simulink library "MyDatacenterModel_GRIDS_HVAC"  (R2025b)
settings: Solver=VariableStepAuto  StartTime=0.0  StopTime=10.0  RelTol=1e-3
libraries: fl_lib x119, datacenter_lib x13, buildingEnergy_lib x11, ee_lib x1
settings Model: Creator=vikrants  LastModifiedBy=skota

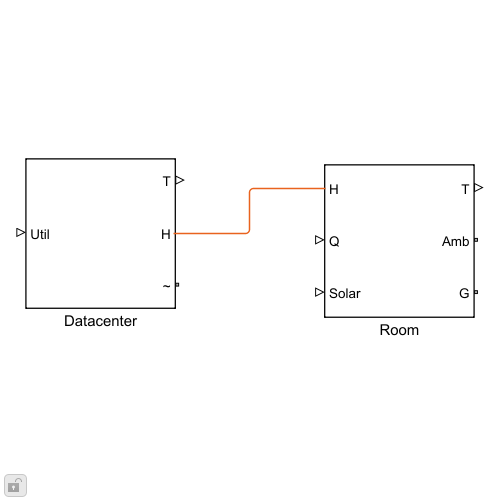
[thumbnail: Simulink's stored preview of the top-level diagram]
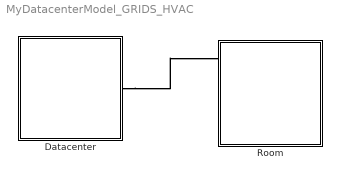
== system MyDatacenterModel_GRIDS_HVAC ==
  Datacenter : Subsystem
  Room : Subsystem
  connections:
  Datacenter/RConn2 -- Room/LConn1

== system MyDatacenterModel_GRIDS_HVAC/Datacenter ==
  Load : ee_lib/Passive/Dynamic Load (Three-Phase)  port_option=ee.enum.threePhasePort.composite  FRated=60 Hz  Vline_rms_min=100 V  tau=0.01 s  Vline_rms_ini=200 V  Vang_ini=0 deg  gmin=0 S
  ServerUnits : Subsystem
  THD : datacenter_lib/Custom Dynamic Load (3-phase) block  Pf=0.98  THD=0  N=12
  Util : PMIOPort  Side=Left
  T : PMIOPort  Port=2  Side=Right
  H : PMIOPort  Port=3  Side=Right
  ~ : PMIOPort  Port=4  Side=Right
  connections:
  ServerUnits/LConn1 -- Util/RConn1
  ServerUnits/RConn2 -- T/RConn1
  ServerUnits/RConn1 -- H/RConn1
  THD/RConn1 -- Load/LConn2
  THD/RConn2 -- Load/LConn3
  THD/LConn1 -- ServerUnits/RConn3
  Load/LConn1 -- ~/RConn1

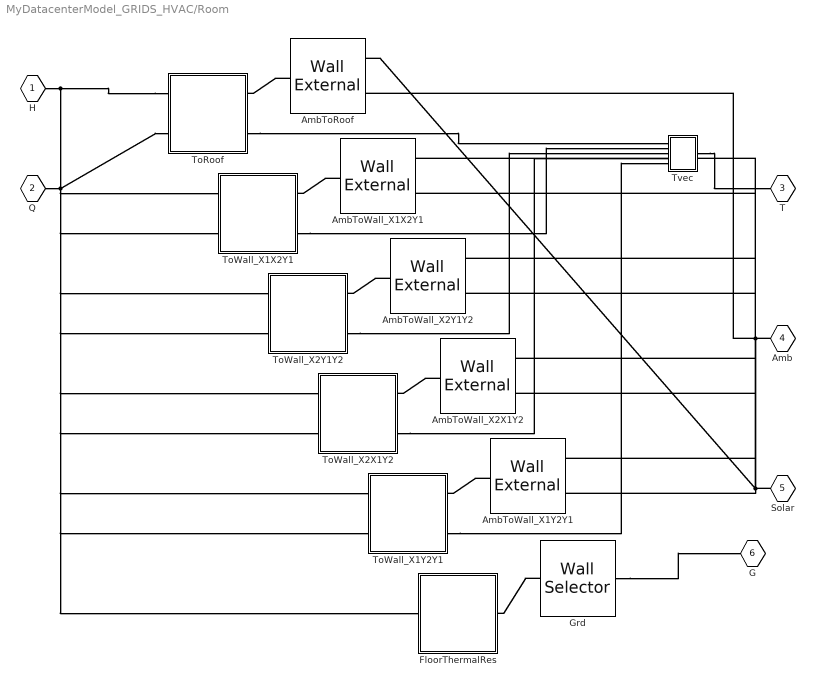
== system MyDatacenterModel_GRIDS_HVAC/Room ==
  AmbToRoof : buildingEnergy_lib/Wall External  extWallModel=wallExternalModelOption.wallSolarWinVent  wallLength=12 m  wallHeight=8 m  wallThickness=0.05 m  wallMaterialDen=4000 kg/m^3  wallMaterialCp=1870 J/(K*kg)  wallAbsorptivity=0.5  wallThermalK=2 W/(K*m)  winLength=1 m  winHeight=0.5 m  winThickness=0.007 m  winMaterialDen=2500 kg/m^3  winMaterialCp=787 J/(K*kg)  winAbsorptivity=0.35  winThermalK=1 W/(K*m)  winTransmissivity=0.45  ventLength=0.1 m  ventHeight=0.1 m  extToWallHTC=5 W/(K*m^2)  intToRoomHTC=5 W/(K*m^2)  iniT=300 K  latitude=5  longitude=5  localTime=5  dayLightS=0  surfAngle=0 deg  surfUnitV="[0.42262    -0.90631]"  startYear=2025  startMonth=1  startDay=1  startHr=1  numHrsData=24  interp_method=simscape.enum.interpolation.linear  extrap_method=simscape.enum.extrapolation.nearest
  AmbToWall_X1X2Y1 : buildingEnergy_lib/Wall External  extWallModel=wallExternalModelOption.wallSolarWinVent  wallLength=12 m  wallHeight=3 m  wallThickness=0.05 m  wallMaterialDen=4000 kg/m^3  wallMaterialCp=1870 J/(K*kg)  wallAbsorptivity=0.5  wallThermalK=2 W/(K*m)  winLength=1 m  winHeight=0.5 m  winThickness=0.007 m  winMaterialDen=2500 kg/m^3  winMaterialCp=787 J/(K*kg)  winAbsorptivity=0.35  winThermalK=1 W/(K*m)  winTransmissivity=0.45  ventLength=0.1 m  ventHeight=0.1 m  extToWallHTC=5 W/(K*m^2)  intToRoomHTC=5 W/(K*m^2)  iniT=300 K  latitude=5  longitude=5  localTime=5  dayLightS=0  surfAngle=90 deg  surfUnitV="[0.42262    -0.90631]"  startYear=2025  startMonth=1  startDay=1  startHr=1  numHrsData=24  interp_method=simscape.enum.interpolation.linear  extrap_method=simscape.enum.extrapolation.nearest
  AmbToWall_X1Y2Y1 : buildingEnergy_lib/Wall External  extWallModel=wallExternalModelOption.wallSolarWinVent  wallLength=8 m  wallHeight=3 m  wallThickness=0.05 m  wallMaterialDen=4000 kg/m^3  wallMaterialCp=1870 J/(K*kg)  wallAbsorptivity=0.5  wallThermalK=2 W/(K*m)  winLength=1 m  winHeight=0.5 m  winThickness=0.007 m  winMaterialDen=2500 kg/m^3  winMaterialCp=787 J/(K*kg)  winAbsorptivity=0.35  winThermalK=1 W/(K*m)  winTransmissivity=0.45  ventLength=0.1 m  ventHeight=0.1 m  extToWallHTC=5 W/(K*m^2)  intToRoomHTC=5 W/(K*m^2)  iniT=300 K  latitude=5  longitude=5  localTime=5  dayLightS=0  surfAngle=90 deg  surfUnitV="[-0.90631    -0.42262]"  startYear=2025  startMonth=1  startDay=1  startHr=1  numHrsData=24  interp_method=simscape.enum.interpolation.linear  extrap_method=simscape.enum.extrapolation.nearest
  AmbToWall_X2X1Y2 : buildingEnergy_lib/Wall External  extWallModel=wallExternalModelOption.wallSolarWinVent  wallLength=12 m  wallHeight=3 m  wallThickness=0.05 m  wallMaterialDen=4000 kg/m^3  wallMaterialCp=1870 J/(K*kg)  wallAbsorptivity=0.5  wallThermalK=2 W/(K*m)  winLength=1 m  winHeight=0.5 m  winThickness=0.007 m  winMaterialDen=2500 kg/m^3  winMaterialCp=787 J/(K*kg)  winAbsorptivity=0.35  winThermalK=1 W/(K*m)  winTransmissivity=0.45  ventLength=0.1 m  ventHeight=0.1 m  extToWallHTC=5 W/(K*m^2)  intToRoomHTC=5 W/(K*m^2)  iniT=300 K  latitude=5  longitude=5  localTime=5  dayLightS=0  surfAngle=90 deg  surfUnitV="[-0.42262     0.90631]"  startYear=2025  startMonth=1  startDay=1  startHr=1  numHrsData=24  interp_method=simscape.enum.interpolation.linear  extrap_method=simscape.enum.extrapolation.nearest
  AmbToWall_X2Y1Y2 : buildingEnergy_lib/Wall External  extWallModel=wallExternalModelOption.wallSolarWinVent  wallLength=8 m  wallHeight=3 m  wallThickness=0.05 m  wallMaterialDen=4000 kg/m^3  wallMaterialCp=1870 J/(K*kg)  wallAbsorptivity=0.5  wallThermalK=2 W/(K*m)  winLength=1 m  winHeight=0.5 m  winThickness=0.007 m  winMaterialDen=2500 kg/m^3  winMaterialCp=787 J/(K*kg)  winAbsorptivity=0.35  winThermalK=1 W/(K*m)  winTransmissivity=0.45  ventLength=0.1 m  ventHeight=0.1 m  extToWallHTC=5 W/(K*m^2)  intToRoomHTC=5 W/(K*m^2)  iniT=300 K  latitude=5  longitude=5  localTime=5  dayLightS=0  surfAngle=90 deg  surfUnitV="[0.90631     0.42262]"  startYear=2025  startMonth=1  startDay=1  startHr=1  numHrsData=24  interp_method=simscape.enum.interpolation.linear  extrap_method=simscape.enum.extrapolation.nearest
  FloorThermalRes : Subsystem
  Grd : buildingEnergy_lib/Wall Selector  optWall=1  wallLength=12 m  wallHeight=8 m  wallThickness=0.05 m  wallMaterialDen=4000 kg/m^3  wallMaterialCp=1870 J/(K*kg)  wallAbsorptivity=0.5  wallThermalK=2 W/(K*m)  winLength=1 m  winHeight=0.5 m  winThickness=0.007 m  winMaterialDen=2500 kg/m^3  winMaterialCp=787 J/(K*kg)  winAbsorptivity=0.35  winThermalK=1 W/(K*m)  winTransmissivity=0.45  ventLength=0.1 m  ventHeight=0.1 m  extToWallHTC=5 W/(K*m^2)  intToRoomHTC=5 W/(K*m^2)  iniT=300 K
  ToRoof : Subsystem
  ToWall_X1X2Y1 : Subsystem
  ToWall_X1Y2Y1 : Subsystem
  ToWall_X2X1Y2 : Subsystem
  ToWall_X2Y1Y2 : Subsystem
  Tvec : Subsystem
  H : PMIOPort  Side=Left
  Q : PMIOPort  Port=2  Side=Left
  T : PMIOPort  Port=3  Side=Right
  Amb : PMIOPort  Port=4  Side=Right
  Solar : PMIOPort  Port=5  Side=Left
  G : PMIOPort  Port=6  Side=Right
  connections:
  ToRoof/LConn1 -- H/RConn1 -- ToWall_X1X2Y1/LConn1 -- ToWall_X2Y1Y2/LConn1 -- ToWall_X2X1Y2/LConn1 -- ToWall_X1Y2Y1/LConn1 -- FloorThermalRes/LConn1
  ToRoof/LConn2 -- Q/RConn1 -- ToWall_X1X2Y1/LConn2 -- ToWall_X2Y1Y2/LConn2 -- ToWall_X2X1Y2/LConn2 -- ToWall_X1Y2Y1/LConn2
  AmbToRoof/RConn1 -- ToRoof/RConn1
  AmbToRoof/LConn2 -- Amb/RConn1 -- AmbToWall_X1X2Y1/LConn2 -- AmbToWall_X2Y1Y2/LConn2 -- AmbToWall_X2X1Y2/LConn2 -- AmbToWall_X1Y2Y1/LConn2
  AmbToRoof/LConn1 -- Solar/RConn1 -- AmbToWall_X1X2Y1/LConn1 -- AmbToWall_X2Y1Y2/LConn1 -- AmbToWall_X2X1Y2/LConn1 -- AmbToWall_X1Y2Y1/LConn1
  ToRoof/RConn2 -- Tvec/LConn1
  AmbToWall_X1X2Y1/RConn1 -- ToWall_X1X2Y1/RConn1
  ToWall_X1X2Y1/RConn2 -- Tvec/LConn2
  AmbToWall_X2Y1Y2/RConn1 -- ToWall_X2Y1Y2/RConn1
  ToWall_X2Y1Y2/RConn2 -- Tvec/LConn3
  AmbToWall_X2X1Y2/RConn1 -- ToWall_X2X1Y2/RConn1
  ToWall_X2X1Y2/RConn2 -- Tvec/LConn4
  AmbToWall_X1Y2Y1/RConn1 -- ToWall_X1Y2Y1/RConn1
  ToWall_X1Y2Y1/RConn2 -- Tvec/LConn5
  Tvec/RConn1 -- T/RConn1
  Grd/LConn1 -- G/RConn1
  Grd/RConn1 -- FloorThermalRes/RConn1

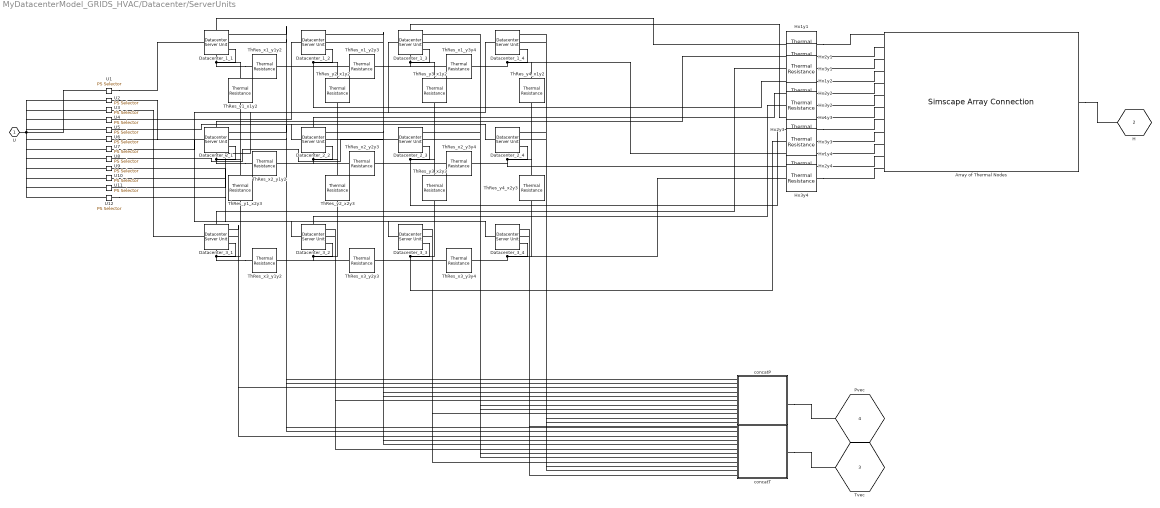
== system MyDatacenterModel_GRIDS_HVAC/Datacenter/ServerUnits ==
  Array of Thermal Nodes : SimscapeArrayConnection  Domain=foundation.thermal.thermal  ConcatenateDimension=1  NumScalarElements=12
  Datacenter_1_{1..4} (4 alike) : datacenter_lib/Datacenter Server Unit  peakPowCPU=40 W  numOfCPU=2  peakPowMemory=9 W  numOfMemory=4  peakPowDisk=12 W  numOfDisk=1  peakPowPCIslot=25 W  numOfPCIslot=2  peakPowMotherboard=25 W  numOfMotherboard=1  peakPowFan=10 W  numOfFan=1  powerSupplyEff=85  numCPUperServer=11  ratioActualToNameplate=0.6  serverMass=50 kg  serverSpHeat=2500 J/(K*kg)  idlePower=25 W  physQ=datacenterPhysics.linear  calibParam=1  T_specify=off  T_priority=High  T=300 K  T_nominal_specify=off  T_nominal_value=1  T_nominal_unit=K  Q_specify=off  Q_priority=None  Q=0 W  Q_nominal_specify=off  Q_nominal_value=1  Q_nominal_unit=W
  Datacenter_2_{1..4} (4 alike) : datacenter_lib/Datacenter Server Unit  peakPowCPU=40 W  numOfCPU=2  peakPowMemory=9 W  numOfMemory=4  peakPowDisk=12 W  numOfDisk=1  peakPowPCIslot=25 W  numOfPCIslot=2  peakPowMotherboard=25 W  numOfMotherboard=1  peakPowFan=10 W  numOfFan=1  powerSupplyEff=85  numCPUperServer=11  ratioActualToNameplate=0.6  serverMass=50 kg  serverSpHeat=2500 J/(K*kg)  idlePower=25 W  physQ=datacenterPhysics.linear  calibParam=1  T_specify=off  T_priority=High  T=300 K  T_nominal_specify=off  T_nominal_value=1  T_nominal_unit=K  Q_specify=off  Q_priority=None  Q=0 W  Q_nominal_specify=off  Q_nominal_value=1  Q_nominal_unit=W
  Datacenter_3_{1..4} (4 alike) : datacenter_lib/Datacenter Server Unit  peakPowCPU=40 W  numOfCPU=2  peakPowMemory=9 W  numOfMemory=4  peakPowDisk=12 W  numOfDisk=1  peakPowPCIslot=25 W  numOfPCIslot=2  peakPowMotherboard=25 W  numOfMotherboard=1  peakPowFan=10 W  numOfFan=1  powerSupplyEff=85  numCPUperServer=11  ratioActualToNameplate=0.6  serverMass=50 kg  serverSpHeat=2500 J/(K*kg)  idlePower=25 W  physQ=datacenterPhysics.linear  calibParam=1  T_specify=off  T_priority=High  T=300 K  T_nominal_specify=off  T_nominal_value=1  T_nominal_unit=K  Q_specify=off  Q_priority=None  Q=0 W  Q_nominal_specify=off  Q_nominal_value=1  Q_nominal_unit=W
  Hx1y{1..4} (4 alike) : fl_lib/Thermal/Thermal Elements/Thermal Resistance  resistance=0.01 K/W  T_specify=off  T_priority=None  T=0 K  T_nominal_specify=off  T_nominal_value=1  T_nominal_unit=K  Q_specify=off  Q_priority=None  Q=0 W  Q_nominal_specify=off  Q_nominal_value=1  Q_nominal_unit=W
  Hx2y{1..4} (4 alike) : fl_lib/Thermal/Thermal Elements/Thermal Resistance  resistance=0.01 K/W  T_specify=off  T_priority=None  T=0 K  T_nominal_specify=off  T_nominal_value=1  T_nominal_unit=K  Q_specify=off  Q_priority=None  Q=0 W  Q_nominal_specify=off  Q_nominal_value=1  Q_nominal_unit=W
  Hx3y{1..4} (4 alike) : fl_lib/Thermal/Thermal Elements/Thermal Resistance  resistance=0.01 K/W  T_specify=off  T_priority=None  T=0 K  T_nominal_specify=off  T_nominal_value=1  T_nominal_unit=K  Q_specify=off  Q_priority=None  Q=0 W  Q_nominal_specify=off  Q_nominal_value=1  Q_nominal_unit=W
  ThRes_x1_y1y2 : fl_lib/Thermal/Thermal Elements/Thermal Resistance  resistance=0.01 K/W  T_specify=off  T_priority=None  T=0 K  T_nominal_specify=off  T_nominal_value=1  T_nominal_unit=K  Q_specify=off  Q_priority=None  Q=0 W  Q_nominal_specify=off  Q_nominal_value=1  Q_nominal_unit=W
  ThRes_x1_y2y3 : fl_lib/Thermal/Thermal Elements/Thermal Resistance  resistance=0.01 K/W  T_specify=off  T_priority=None  T=0 K  T_nominal_specify=off  T_nominal_value=1  T_nominal_unit=K  Q_specify=off  Q_priority=None  Q=0 W  Q_nominal_specify=off  Q_nominal_value=1  Q_nominal_unit=W
  ThRes_x1_y3y4 : fl_lib/Thermal/Thermal Elements/Thermal Resistance  resistance=0.01 K/W  T_specify=off  T_priority=None  T=0 K  T_nominal_specify=off  T_nominal_value=1  T_nominal_unit=K  Q_specify=off  Q_priority=None  Q=0 W  Q_nominal_specify=off  Q_nominal_value=1  Q_nominal_unit=W
  ThRes_x2_y1y2 : fl_lib/Thermal/Thermal Elements/Thermal Resistance  resistance=0.01 K/W  T_specify=off  T_priority=None  T=0 K  T_nominal_specify=off  T_nominal_value=1  T_nominal_unit=K  Q_specify=off  Q_priority=None  Q=0 W  Q_nominal_specify=off  Q_nominal_value=1  Q_nominal_unit=W
  ThRes_x2_y2y3 : fl_lib/Thermal/Thermal Elements/Thermal Resistance  resistance=0.01 K/W  T_specify=off  T_priority=None  T=0 K  T_nominal_specify=off  T_nominal_value=1  T_nominal_unit=K  Q_specify=off  Q_priority=None  Q=0 W  Q_nominal_specify=off  Q_nominal_value=1  Q_nominal_unit=W
  ThRes_x2_y3y4 : fl_lib/Thermal/Thermal Elements/Thermal Resistance  resistance=0.01 K/W  T_specify=off  T_priority=None  T=0 K  T_nominal_specify=off  T_nominal_value=1  T_nominal_unit=K  Q_specify=off  Q_priority=None  Q=0 W  Q_nominal_specify=off  Q_nominal_value=1  Q_nominal_unit=W
  ThRes_x3_y1y2 : fl_lib/Thermal/Thermal Elements/Thermal Resistance  resistance=0.01 K/W  T_specify=off  T_priority=None  T=0 K  T_nominal_specify=off  T_nominal_value=1  T_nominal_unit=K  Q_specify=off  Q_priority=None  Q=0 W  Q_nominal_specify=off  Q_nominal_value=1  Q_nominal_unit=W
  ThRes_x3_y2y3 : fl_lib/Thermal/Thermal Elements/Thermal Resistance  resistance=0.01 K/W  T_specify=off  T_priority=None  T=0 K  T_nominal_specify=off  T_nominal_value=1  T_nominal_unit=K  Q_specify=off  Q_priority=None  Q=0 W  Q_nominal_specify=off  Q_nominal_value=1  Q_nominal_unit=W
  ThRes_x3_y3y4 : fl_lib/Thermal/Thermal Elements/Thermal Resistance  resistance=0.01 K/W  T_specify=off  T_priority=None  T=0 K  T_nominal_specify=off  T_nominal_value=1  T_nominal_unit=K  Q_specify=off  Q_priority=None  Q=0 W  Q_nominal_specify=off  Q_nominal_value=1  Q_nominal_unit=W
  ThRes_y1_x1y2 : fl_lib/Thermal/Thermal Elements/Thermal Resistance  resistance=0.01 K/W  T_specify=off  T_priority=None  T=0 K  T_nominal_specify=off  T_nominal_value=1  T_nominal_unit=K  Q_specify=off  Q_priority=None  Q=0 W  Q_nominal_specify=off  Q_nominal_value=1  Q_nominal_unit=W
  ThRes_y1_x2y3 : fl_lib/Thermal/Thermal Elements/Thermal Resistance  resistance=0.01 K/W  T_specify=off  T_priority=None  T=0 K  T_nominal_specify=off  T_nominal_value=1  T_nominal_unit=K  Q_specify=off  Q_priority=None  Q=0 W  Q_nominal_specify=off  Q_nominal_value=1  Q_nominal_unit=W
  ThRes_y2_x1y2 : fl_lib/Thermal/Thermal Elements/Thermal Resistance  resistance=0.01 K/W  T_specify=off  T_priority=None  T=0 K  T_nominal_specify=off  T_nominal_value=1  T_nominal_unit=K  Q_specify=off  Q_priority=None  Q=0 W  Q_nominal_specify=off  Q_nominal_value=1  Q_nominal_unit=W
  ThRes_y2_x2y3 : fl_lib/Thermal/Thermal Elements/Thermal Resistance  resistance=0.01 K/W  T_specify=off  T_priority=None  T=0 K  T_nominal_specify=off  T_nominal_value=1  T_nominal_unit=K  Q_specify=off  Q_priority=None  Q=0 W  Q_nominal_specify=off  Q_nominal_value=1  Q_nominal_unit=W
  ThRes_y3_x1y2 : fl_lib/Thermal/Thermal Elements/Thermal Resistance  resistance=0.01 K/W  T_specify=off  T_priority=None  T=0 K  T_nominal_specify=off  T_nominal_value=1  T_nominal_unit=K  Q_specify=off  Q_priority=None  Q=0 W  Q_nominal_specify=off  Q_nominal_value=1  Q_nominal_unit=W
  ThRes_y3_x2y3 : fl_lib/Thermal/Thermal Elements/Thermal Resistance  resistance=0.01 K/W  T_specify=off  T_priority=None  T=0 K  T_nominal_specify=off  T_nominal_value=1  T_nominal_unit=K  Q_specify=off  Q_priority=None  Q=0 W  Q_nominal_specify=off  Q_nominal_value=1  Q_nominal_unit=W
  ThRes_y4_x1y2 : fl_lib/Thermal/Thermal Elements/Thermal Resistance  resistance=0.01 K/W  T_specify=off  T_priority=None  T=0 K  T_nominal_specify=off  T_nominal_value=1  T_nominal_unit=K  Q_specify=off  Q_priority=None  Q=0 W  Q_nominal_specify=off  Q_nominal_value=1  Q_nominal_unit=W
  ThRes_y4_x2y3 : fl_lib/Thermal/Thermal Elements/Thermal Resistance  resistance=0.01 K/W  T_specify=off  T_priority=None  T=0 K  T_nominal_specify=off  T_nominal_value=1  T_nominal_unit=K  Q_specify=off  Q_priority=None  Q=0 W  Q_nominal_specify=off  Q_nominal_value=1  Q_nominal_unit=W
  U1 : fl_lib/Physical Signals/Nonlinear Operators/PS Selector  ix=1
  U10 : fl_lib/Physical Signals/Nonlinear Operators/PS Selector  ix=10
  U11 : fl_lib/Physical Signals/Nonlinear Operators/PS Selector  ix=11
  U12 : fl_lib/Physical Signals/Nonlinear Operators/PS Selector  ix=12
  U2 : fl_lib/Physical Signals/Nonlinear Operators/PS Selector  ix=2
  U3 : fl_lib/Physical Signals/Nonlinear Operators/PS Selector  ix=3
  U4 : fl_lib/Physical Signals/Nonlinear Operators/PS Selector  ix=4
  U5 : fl_lib/Physical Signals/Nonlinear Operators/PS Selector  ix=5
  U6 : fl_lib/Physical Signals/Nonlinear Operators/PS Selector  ix=6
  U7 : fl_lib/Physical Signals/Nonlinear Operators/PS Selector  ix=7
  U8 : fl_lib/Physical Signals/Nonlinear Operators/PS Selector  ix=8
  U9 : fl_lib/Physical Signals/Nonlinear Operators/PS Selector  ix=9
  concatP : Subsystem
  concatT : Subsystem
  U : PMIOPort  Side=Left
  H : PMIOPort  Port=2  Side=Right
  Tvec : PMIOPort  Port=3  Side=Right
  Pvec : PMIOPort  Port=4  Side=Right
  connections:
  ThRes_x1_y1y2/LConn1 -- Datacenter_1_1/RConn3 -- ThRes_y1_x1y2/LConn1 -- Hx1y1/LConn1
  ThRes_x1_y1y2/RConn1 -- Datacenter_1_2/RConn3 -- ThRes_x1_y2y3/LConn1 -- ThRes_y2_x1y2/LConn1 -- Hx1y2/LConn1
  ThRes_x1_y2y3/RConn1 -- Datacenter_1_3/RConn3 -- ThRes_x1_y3y4/LConn1 -- ThRes_y3_x1y2/LConn1 -- Hx1y3/LConn1
  ThRes_x1_y3y4/RConn1 -- Datacenter_1_4/RConn3 -- ThRes_y4_x1y2/LConn1 -- Hx1y4/LConn1
  ThRes_x2_y1y2/LConn1 -- Datacenter_2_1/RConn3 -- ThRes_y1_x1y2/RConn1 -- ThRes_y1_x2y3/LConn1 -- Hx2y1/LConn1
  ThRes_x2_y1y2/RConn1 -- Datacenter_2_2/RConn3 -- ThRes_x2_y2y3/LConn1 -- ThRes_y2_x1y2/RConn1 -- ThRes_y2_x2y3/LConn1 -- Hx2y2/LConn1
  ThRes_x2_y2y3/RConn1 -- Datacenter_2_3/RConn3 -- ThRes_x2_y3y4/LConn1 -- ThRes_y3_x1y2/RConn1 -- ThRes_y3_x2y3/LConn1 -- Hx2y3/LConn1
  ThRes_x2_y3y4/RConn1 -- Datacenter_2_4/RConn3 -- ThRes_y4_x1y2/RConn1 -- ThRes_y4_x2y3/LConn1 -- Hx2y4/LConn1
  ThRes_x3_y1y2/LConn1 -- Datacenter_3_1/RConn3 -- ThRes_y1_x2y3/RConn1 -- Hx3y1/LConn1
  ThRes_x3_y1y2/RConn1 -- Datacenter_3_2/RConn3 -- ThRes_x3_y2y3/LConn1 -- ThRes_y2_x2y3/RConn1 -- Hx3y2/LConn1
  ThRes_x3_y2y3/RConn1 -- Datacenter_3_3/RConn3 -- ThRes_x3_y3y4/LConn1 -- ThRes_y3_x2y3/RConn1 -- Hx3y3/LConn1
  ThRes_x3_y3y4/RConn1 -- Datacenter_3_4/RConn3 -- ThRes_y4_x2y3/RConn1 -- Hx3y4/LConn1
  U1/LConn1 -- U2/LConn1 -- U3/LConn1 -- U4/LConn1 -- U5/LConn1 -- U6/LConn1 -- U7/LConn1 -- U8/LConn1 -- U9/LConn1 -- U10/LConn1 -- U11/LConn1 -- U/RConn1 -- U12/LConn1
  U1/RConn1 -- Datacenter_1_1/LConn1
  U2/RConn1 -- Datacenter_2_1/LConn1
  U3/RConn1 -- Datacenter_3_1/LConn1
  U4/RConn1 -- Datacenter_1_2/LConn1
  U5/RConn1 -- Datacenter_2_2/LConn1
  U6/RConn1 -- Datacenter_3_2/LConn1
  U7/RConn1 -- Datacenter_1_3/LConn1
  U8/RConn1 -- Datacenter_2_3/LConn1
  U9/RConn1 -- Datacenter_3_3/LConn1
  U10/RConn1 -- Datacenter_1_4/LConn1
  U11/RConn1 -- Datacenter_2_4/LConn1
  U12/RConn1 -- Datacenter_3_4/LConn1
  Array of Thermal Nodes/RConn1 -- H/RConn1
  Hx1y1/RConn1 -- Array of Thermal Nodes/LConn1
  Hx2y1/RConn1 -- Array of Thermal Nodes/LConn2
  Hx3y1/RConn1 -- Array of Thermal Nodes/LConn3
  Hx1y2/RConn1 -- Array of Thermal Nodes/LConn4
  Hx2y2/RConn1 -- Array of Thermal Nodes/LConn5
  Hx3y2/RConn1 -- Array of Thermal Nodes/LConn6
  Hx1y3/RConn1 -- Array of Thermal Nodes/LConn7
  Hx2y3/RConn1 -- Array of Thermal Nodes/LConn8
  Hx3y3/RConn1 -- Array of Thermal Nodes/LConn9
  Hx1y4/RConn1 -- Array of Thermal Nodes/LConn10
  Hx2y4/RConn1 -- Array of Thermal Nodes/LConn11
  Hx3y4/RConn1 -- Array of Thermal Nodes/LConn12
  concatT/RConn1 -- Tvec/RConn1
  concatT/LConn1 -- Datacenter_1_1/RConn1
  concatT/LConn2 -- Datacenter_2_1/RConn1
  concatT/LConn3 -- Datacenter_3_1/RConn1
  concatT/LConn4 -- Datacenter_1_2/RConn1
  concatT/LConn5 -- Datacenter_2_2/RConn1
  concatT/LConn6 -- Datacenter_3_2/RConn1
  concatT/LConn7 -- Datacenter_1_3/RConn1
  concatT/LConn8 -- Datacenter_2_3/RConn1
  concatT/LConn9 -- Datacenter_3_3/RConn1
  concatT/LConn10 -- Datacenter_1_4/RConn1
  concatT/LConn11 -- Datacenter_2_4/RConn1
  concatT/LConn12 -- Datacenter_3_4/RConn1
  concatP/RConn1 -- Pvec/RConn1
  concatP/LConn1 -- Datacenter_1_1/RConn2
  concatP/LConn2 -- Datacenter_2_1/RConn2
  concatP/LConn3 -- Datacenter_3_1/RConn2
  concatP/LConn4 -- Datacenter_1_2/RConn2
  concatP/LConn5 -- Datacenter_2_2/RConn2
  concatP/LConn6 -- Datacenter_3_2/RConn2
  concatP/LConn7 -- Datacenter_1_3/RConn2
  concatP/LConn8 -- Datacenter_2_3/RConn2
  concatP/LConn9 -- Datacenter_3_3/RConn2
  concatP/LConn10 -- Datacenter_1_4/RConn2
  concatP/LConn11 -- Datacenter_2_4/RConn2
  concatP/LConn12 -- Datacenter_3_4/RConn2

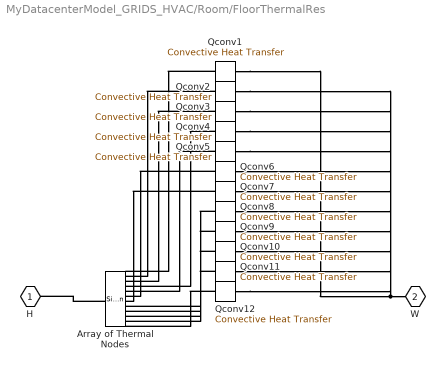
== system MyDatacenterModel_GRIDS_HVAC/Room/FloorThermalRes ==
  Array of Thermal Nodes : SimscapeArrayConnection  Domain=foundation.thermal.thermal  ConcatenateDimension=1  NumScalarElements=12
  Qconv{1..12} (12 alike) : fl_lib/Thermal/Thermal Elements/Convective Heat Transfer  thermal_type=foundation.enum.constant_variable.constant  area=8 m^2  heat_tr_coeff=20 W/(K*m^2)  min_heat_tr_coeff=1e-3 W/(K*m^2)  T_specify=off  T_priority=None  T=0 K  T_nominal_specify=off  T_nominal_value=1  T_nominal_unit=K  Q_specify=off  Q_priority=None  Q=0 W  Q_nominal_specify=off  Q_nominal_value=1  Q_nominal_unit=W
  H : PMIOPort  Side=Left
  W : PMIOPort  Port=2  Side=Right
  connections:
  Array of Thermal Nodes/RConn1 -- H/RConn1
  Qconv1/LConn1 -- Array of Thermal Nodes/LConn1
  Qconv1/RConn1 -- Qconv2/RConn1 -- Qconv3/RConn1 -- Qconv4/RConn1 -- Qconv5/RConn1 -- Qconv6/RConn1 -- Qconv7/RConn1 -- Qconv8/RConn1 -- Qconv9/RConn1 -- Qconv10/RConn1 -- Qconv11/RConn1 -- W/RConn1 -- Qconv12/RConn1
  Qconv2/LConn1 -- Array of Thermal Nodes/LConn2
  Qconv3/LConn1 -- Array of Thermal Nodes/LConn3
  Qconv4/LConn1 -- Array of Thermal Nodes/LConn4
  Qconv5/LConn1 -- Array of Thermal Nodes/LConn5
  Qconv6/LConn1 -- Array of Thermal Nodes/LConn6
  Qconv7/LConn1 -- Array of Thermal Nodes/LConn7
  Qconv8/LConn1 -- Array of Thermal Nodes/LConn8
  Qconv9/LConn1 -- Array of Thermal Nodes/LConn9
  Qconv10/LConn1 -- Array of Thermal Nodes/LConn10
  Qconv11/LConn1 -- Array of Thermal Nodes/LConn11
  Qconv12/LConn1 -- Array of Thermal Nodes/LConn12

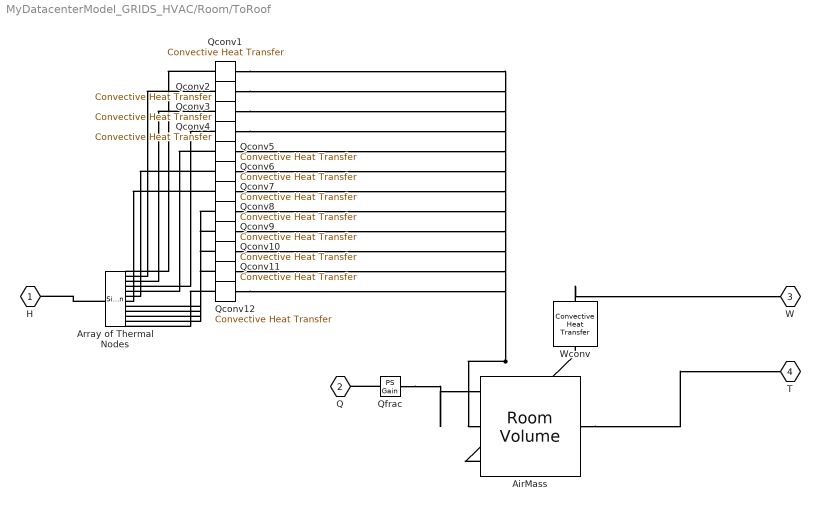
== system MyDatacenterModel_GRIDS_HVAC/Room/ToRoof ==
  AirMass : buildingEnergy_lib/Room Volume  N1=1  N2=1  iniT=300 K  length=12 m  width=8 m  height=0.10667 m
  Array of Thermal Nodes : SimscapeArrayConnection  Domain=foundation.thermal.thermal  ConcatenateDimension=1  NumScalarElements=12
  Qconv{1..12} (12 alike) : fl_lib/Thermal/Thermal Elements/Convective Heat Transfer  thermal_type=foundation.enum.constant_variable.constant  area=8 m^2  heat_tr_coeff=20 W/(K*m^2)  min_heat_tr_coeff=1e-3 W/(K*m^2)  T_specify=off  T_priority=None  T=0 K  T_nominal_specify=off  T_nominal_value=1  T_nominal_unit=K  Q_specify=off  Q_priority=None  Q=0 W  Q_nominal_specify=off  Q_nominal_value=1  Q_nominal_unit=W
  Qfrac : fl_lib/Physical Signals/Functions/PS Gain  gain=0.44444
  Wconv : fl_lib/Thermal/Thermal Elements/Convective Heat Transfer  thermal_type=foundation.enum.constant_variable.constant  area=96 m^2  heat_tr_coeff=20 W/(K*m^2)  min_heat_tr_coeff=1e-3 W/(K*m^2)  T_specify=off  T_priority=None  T=0 K  T_nominal_specify=off  T_nominal_value=1  T_nominal_unit=K  Q_specify=off  Q_priority=None  Q=0 W  Q_nominal_specify=off  Q_nominal_value=1  Q_nominal_unit=W
  H : PMIOPort  Side=Left
  Q : PMIOPort  Port=2  Side=Left
  W : PMIOPort  Port=3  Side=Right
  T : PMIOPort  Port=4  Side=Right
  connections:
  Array of Thermal Nodes/RConn1 -- H/RConn1
  Qfrac/LConn1 -- Q/RConn1
  Qfrac/RConn1 -- AirMass/LConn1
  AirMass/LConn3 -- Wconv/LConn1
  Wconv/RConn1 -- W/RConn1
  AirMass/RConn1 -- T/RConn1
  Qconv1/LConn1 -- Array of Thermal Nodes/LConn1
  Qconv1/RConn1 -- Qconv2/RConn1 -- Qconv3/RConn1 -- Qconv4/RConn1 -- Qconv5/RConn1 -- Qconv6/RConn1 -- Qconv7/RConn1 -- Qconv8/RConn1 -- Qconv9/RConn1 -- Qconv10/RConn1 -- Qconv11/RConn1 -- AirMass/LConn2 -- Qconv12/RConn1
  Qconv2/LConn1 -- Array of Thermal Nodes/LConn2
  Qconv3/LConn1 -- Array of Thermal Nodes/LConn3
  Qconv4/LConn1 -- Array of Thermal Nodes/LConn4
  Qconv5/LConn1 -- Array of Thermal Nodes/LConn5
  Qconv6/LConn1 -- Array of Thermal Nodes/LConn6
  Qconv7/LConn1 -- Array of Thermal Nodes/LConn7
  Qconv8/LConn1 -- Array of Thermal Nodes/LConn8
  Qconv9/LConn1 -- Array of Thermal Nodes/LConn9
  Qconv10/LConn1 -- Array of Thermal Nodes/LConn10
  Qconv11/LConn1 -- Array of Thermal Nodes/LConn11
  Qconv12/LConn1 -- Array of Thermal Nodes/LConn12

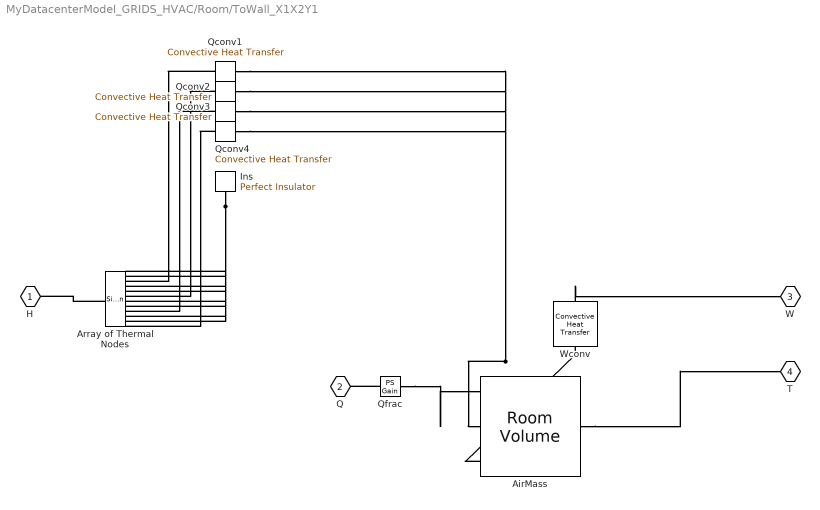
== system MyDatacenterModel_GRIDS_HVAC/Room/ToWall_X1X2Y1 ==
  AirMass : buildingEnergy_lib/Room Volume  N1=1  N2=1  iniT=300 K  length=12 m  width=0.10667 m  height=8 m
  Array of Thermal Nodes : SimscapeArrayConnection  Domain=foundation.thermal.thermal  ConcatenateDimension=1  NumScalarElements=12
  Ins : fl_lib/Thermal/Thermal Elements/Perfect Insulator  T_specify=off  T_priority=None  T=293.15 K  T_nominal_specify=off  T_nominal_value=1  T_nominal_unit=K
  Qconv{1..4} (4 alike) : fl_lib/Thermal/Thermal Elements/Convective Heat Transfer  thermal_type=foundation.enum.constant_variable.constant  area=12 m^2  heat_tr_coeff=20 W/(K*m^2)  min_heat_tr_coeff=1e-3 W/(K*m^2)  T_specify=off  T_priority=None  T=0 K  T_nominal_specify=off  T_nominal_value=1  T_nominal_unit=K  Q_specify=off  Q_priority=None  Q=0 W  Q_nominal_specify=off  Q_nominal_value=1  Q_nominal_unit=W
  Qfrac : fl_lib/Physical Signals/Functions/PS Gain  gain=0.16667
  Wconv : fl_lib/Thermal/Thermal Elements/Convective Heat Transfer  thermal_type=foundation.enum.constant_variable.constant  area=36 m^2  heat_tr_coeff=20 W/(K*m^2)  min_heat_tr_coeff=1e-3 W/(K*m^2)  T_specify=off  T_priority=None  T=0 K  T_nominal_specify=off  T_nominal_value=1  T_nominal_unit=K  Q_specify=off  Q_priority=None  Q=0 W  Q_nominal_specify=off  Q_nominal_value=1  Q_nominal_unit=W
  H : PMIOPort  Side=Left
  Q : PMIOPort  Port=2  Side=Left
  W : PMIOPort  Port=3  Side=Right
  T : PMIOPort  Port=4  Side=Right
  connections:
  Array of Thermal Nodes/RConn1 -- H/RConn1
  Qfrac/LConn1 -- Q/RConn1
  Qfrac/RConn1 -- AirMass/LConn1
  AirMass/LConn3 -- Wconv/LConn1
  Wconv/RConn1 -- W/RConn1
  AirMass/RConn1 -- T/RConn1
  Qconv1/LConn1 -- Array of Thermal Nodes/LConn3
  Qconv1/RConn1 -- Qconv2/RConn1 -- Qconv3/RConn1 -- AirMass/LConn2 -- Qconv4/RConn1
  Qconv2/LConn1 -- Array of Thermal Nodes/LConn6
  Qconv3/LConn1 -- Array of Thermal Nodes/LConn9
  Qconv4/LConn1 -- Array of Thermal Nodes/LConn12
  Array of Thermal Nodes/LConn1 -- Ins/LConn1 -- Array of Thermal Nodes/LConn2 -- Array of Thermal Nodes/LConn4 -- Array of Thermal Nodes/LConn5 -- Array of Thermal Nodes/LConn7 -- Array of Thermal Nodes/LConn8 -- Array of Thermal Nodes/LConn10 -- Array of Thermal Nodes/LConn11

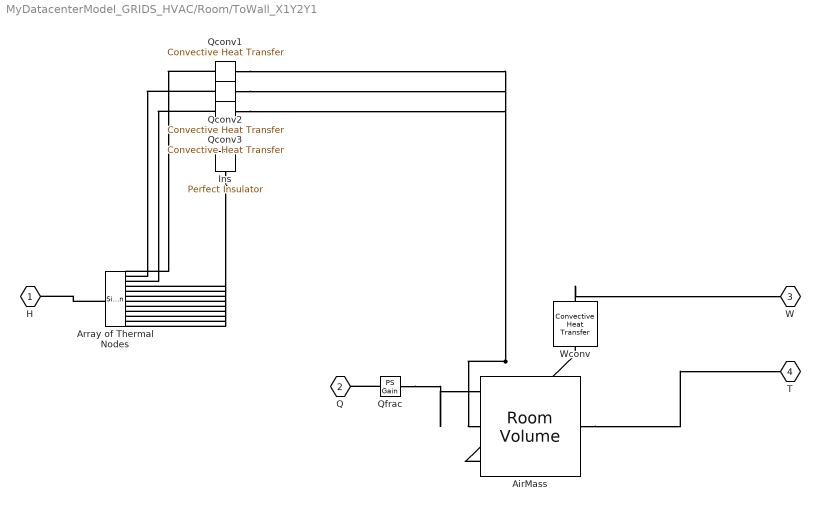
== system MyDatacenterModel_GRIDS_HVAC/Room/ToWall_X1Y2Y1 ==
  AirMass : buildingEnergy_lib/Room Volume  N1=1  N2=1  iniT=300 K  length=8 m  width=0.10667 m  height=3 m
  Array of Thermal Nodes : SimscapeArrayConnection  Domain=foundation.thermal.thermal  ConcatenateDimension=1  NumScalarElements=12
  Ins : fl_lib/Thermal/Thermal Elements/Perfect Insulator  T_specify=off  T_priority=None  T=293.15 K  T_nominal_specify=off  T_nominal_value=1  T_nominal_unit=K
  Qconv1 : fl_lib/Thermal/Thermal Elements/Convective Heat Transfer  thermal_type=foundation.enum.constant_variable.constant  area=6 m^2  heat_tr_coeff=20 W/(K*m^2)  min_heat_tr_coeff=1e-3 W/(K*m^2)  T_specify=off  T_priority=None  T=0 K  T_nominal_specify=off  T_nominal_value=1  T_nominal_unit=K  Q_specify=off  Q_priority=None  Q=0 W  Q_nominal_specify=off  Q_nominal_value=1  Q_nominal_unit=W
  Qconv2 : fl_lib/Thermal/Thermal Elements/Convective Heat Transfer  thermal_type=foundation.enum.constant_variable.constant  area=6 m^2  heat_tr_coeff=20 W/(K*m^2)  min_heat_tr_coeff=1e-3 W/(K*m^2)  T_specify=off  T_priority=None  T=0 K  T_nominal_specify=off  T_nominal_value=1  T_nominal_unit=K  Q_specify=off  Q_priority=None  Q=0 W  Q_nominal_specify=off  Q_nominal_value=1  Q_nominal_unit=W
  Qconv3 : fl_lib/Thermal/Thermal Elements/Convective Heat Transfer  thermal_type=foundation.enum.constant_variable.constant  area=6 m^2  heat_tr_coeff=20 W/(K*m^2)  min_heat_tr_coeff=1e-3 W/(K*m^2)  T_specify=off  T_priority=None  T=0 K  T_nominal_specify=off  T_nominal_value=1  T_nominal_unit=K  Q_specify=off  Q_priority=None  Q=0 W  Q_nominal_specify=off  Q_nominal_value=1  Q_nominal_unit=W
  Qfrac : fl_lib/Physical Signals/Functions/PS Gain  gain=0.11111
  Wconv : fl_lib/Thermal/Thermal Elements/Convective Heat Transfer  thermal_type=foundation.enum.constant_variable.constant  area=24 m^2  heat_tr_coeff=20 W/(K*m^2)  min_heat_tr_coeff=1e-3 W/(K*m^2)  T_specify=off  T_priority=None  T=0 K  T_nominal_specify=off  T_nominal_value=1  T_nominal_unit=K  Q_specify=off  Q_priority=None  Q=0 W  Q_nominal_specify=off  Q_nominal_value=1  Q_nominal_unit=W
  H : PMIOPort  Side=Left
  Q : PMIOPort  Port=2  Side=Left
  W : PMIOPort  Port=3  Side=Right
  T : PMIOPort  Port=4  Side=Right
  connections:
  Array of Thermal Nodes/RConn1 -- H/RConn1
  Qfrac/LConn1 -- Q/RConn1
  Qfrac/RConn1 -- AirMass/LConn1
  AirMass/LConn3 -- Wconv/LConn1
  Wconv/RConn1 -- W/RConn1
  AirMass/RConn1 -- T/RConn1
  Qconv1/LConn1 -- Array of Thermal Nodes/LConn1
  Qconv1/RConn1 -- Qconv2/RConn1 -- AirMass/LConn2 -- Qconv3/RConn1
  Qconv2/LConn1 -- Array of Thermal Nodes/LConn2
  Qconv3/LConn1 -- Array of Thermal Nodes/LConn3
  Array of Thermal Nodes/LConn4 -- Ins/LConn1 -- Array of Thermal Nodes/LConn5 -- Array of Thermal Nodes/LConn6 -- Array of Thermal Nodes/LConn7 -- Array of Thermal Nodes/LConn8 -- Array of Thermal Nodes/LConn9 -- Array of Thermal Nodes/LConn10 -- Array of Thermal Nodes/LConn11 -- Array of Thermal Nodes/LConn12

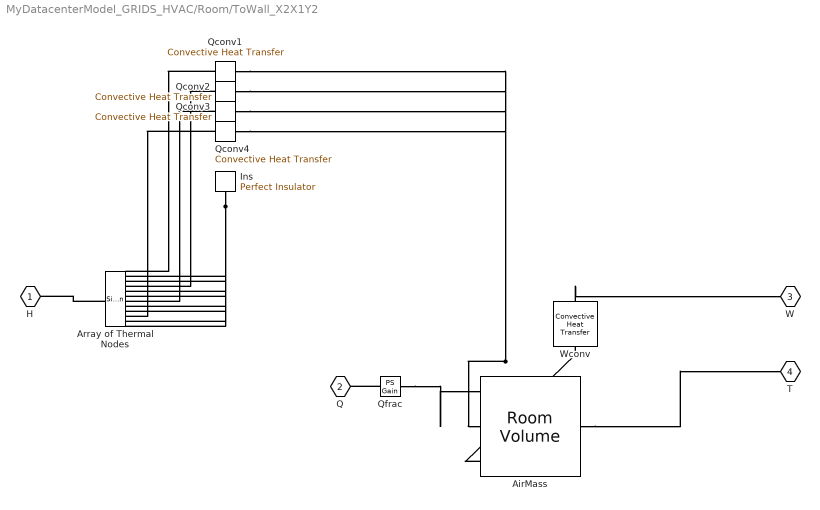
== system MyDatacenterModel_GRIDS_HVAC/Room/ToWall_X2X1Y2 ==
  AirMass : buildingEnergy_lib/Room Volume  N1=1  N2=1  iniT=300 K  length=12 m  width=0.10667 m  height=3 m
  Array of Thermal Nodes : SimscapeArrayConnection  Domain=foundation.thermal.thermal  ConcatenateDimension=1  NumScalarElements=12
  Ins : fl_lib/Thermal/Thermal Elements/Perfect Insulator  T_specify=off  T_priority=None  T=293.15 K  T_nominal_specify=off  T_nominal_value=1  T_nominal_unit=K
  Qconv{1..4} (4 alike) : fl_lib/Thermal/Thermal Elements/Convective Heat Transfer  thermal_type=foundation.enum.constant_variable.constant  area=12 m^2  heat_tr_coeff=20 W/(K*m^2)  min_heat_tr_coeff=1e-3 W/(K*m^2)  T_specify=off  T_priority=None  T=0 K  T_nominal_specify=off  T_nominal_value=1  T_nominal_unit=K  Q_specify=off  Q_priority=None  Q=0 W  Q_nominal_specify=off  Q_nominal_value=1  Q_nominal_unit=W
  Qfrac : fl_lib/Physical Signals/Functions/PS Gain  gain=0.16667
  Wconv : fl_lib/Thermal/Thermal Elements/Convective Heat Transfer  thermal_type=foundation.enum.constant_variable.constant  area=36 m^2  heat_tr_coeff=20 W/(K*m^2)  min_heat_tr_coeff=1e-3 W/(K*m^2)  T_specify=off  T_priority=None  T=0 K  T_nominal_specify=off  T_nominal_value=1  T_nominal_unit=K  Q_specify=off  Q_priority=None  Q=0 W  Q_nominal_specify=off  Q_nominal_value=1  Q_nominal_unit=W
  H : PMIOPort  Side=Left
  Q : PMIOPort  Port=2  Side=Left
  W : PMIOPort  Port=3  Side=Right
  T : PMIOPort  Port=4  Side=Right
  connections:
  Array of Thermal Nodes/RConn1 -- H/RConn1
  Qfrac/LConn1 -- Q/RConn1
  Qfrac/RConn1 -- AirMass/LConn1
  AirMass/LConn3 -- Wconv/LConn1
  Wconv/RConn1 -- W/RConn1
  AirMass/RConn1 -- T/RConn1
  Qconv1/LConn1 -- Array of Thermal Nodes/LConn1
  Qconv1/RConn1 -- Qconv2/RConn1 -- Qconv3/RConn1 -- AirMass/LConn2 -- Qconv4/RConn1
  Qconv2/LConn1 -- Array of Thermal Nodes/LConn4
  Qconv3/LConn1 -- Array of Thermal Nodes/LConn7
  Qconv4/LConn1 -- Array of Thermal Nodes/LConn10
  Array of Thermal Nodes/LConn2 -- Ins/LConn1 -- Array of Thermal Nodes/LConn3 -- Array of Thermal Nodes/LConn5 -- Array of Thermal Nodes/LConn6 -- Array of Thermal Nodes/LConn8 -- Array of Thermal Nodes/LConn9 -- Array of Thermal Nodes/LConn11 -- Array of Thermal Nodes/LConn12

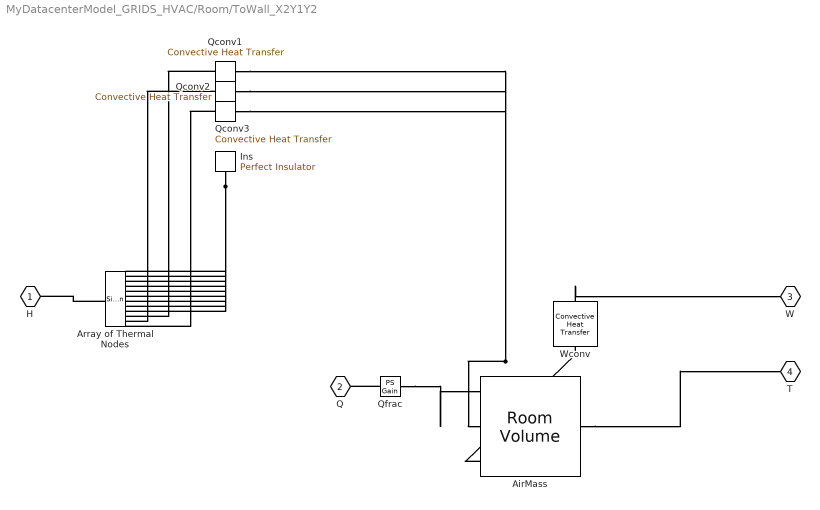
== system MyDatacenterModel_GRIDS_HVAC/Room/ToWall_X2Y1Y2 ==
  AirMass : buildingEnergy_lib/Room Volume  N1=1  N2=1  iniT=300 K  length=8 m  width=0.10667 m  height=3 m
  Array of Thermal Nodes : SimscapeArrayConnection  Domain=foundation.thermal.thermal  ConcatenateDimension=1  NumScalarElements=12
  Ins : fl_lib/Thermal/Thermal Elements/Perfect Insulator  T_specify=off  T_priority=None  T=293.15 K  T_nominal_specify=off  T_nominal_value=1  T_nominal_unit=K
  Qconv1 : fl_lib/Thermal/Thermal Elements/Convective Heat Transfer  thermal_type=foundation.enum.constant_variable.constant  area=6 m^2  heat_tr_coeff=20 W/(K*m^2)  min_heat_tr_coeff=1e-3 W/(K*m^2)  T_specify=off  T_priority=None  T=0 K  T_nominal_specify=off  T_nominal_value=1  T_nominal_unit=K  Q_specify=off  Q_priority=None  Q=0 W  Q_nominal_specify=off  Q_nominal_value=1  Q_nominal_unit=W
  Qconv2 : fl_lib/Thermal/Thermal Elements/Convective Heat Transfer  thermal_type=foundation.enum.constant_variable.constant  area=6 m^2  heat_tr_coeff=20 W/(K*m^2)  min_heat_tr_coeff=1e-3 W/(K*m^2)  T_specify=off  T_priority=None  T=0 K  T_nominal_specify=off  T_nominal_value=1  T_nominal_unit=K  Q_specify=off  Q_priority=None  Q=0 W  Q_nominal_specify=off  Q_nominal_value=1  Q_nominal_unit=W
  Qconv3 : fl_lib/Thermal/Thermal Elements/Convective Heat Transfer  thermal_type=foundation.enum.constant_variable.constant  area=6 m^2  heat_tr_coeff=20 W/(K*m^2)  min_heat_tr_coeff=1e-3 W/(K*m^2)  T_specify=off  T_priority=None  T=0 K  T_nominal_specify=off  T_nominal_value=1  T_nominal_unit=K  Q_specify=off  Q_priority=None  Q=0 W  Q_nominal_specify=off  Q_nominal_value=1  Q_nominal_unit=W
  Qfrac : fl_lib/Physical Signals/Functions/PS Gain  gain=0.11111
  Wconv : fl_lib/Thermal/Thermal Elements/Convective Heat Transfer  thermal_type=foundation.enum.constant_variable.constant  area=24 m^2  heat_tr_coeff=20 W/(K*m^2)  min_heat_tr_coeff=1e-3 W/(K*m^2)  T_specify=off  T_priority=None  T=0 K  T_nominal_specify=off  T_nominal_value=1  T_nominal_unit=K  Q_specify=off  Q_priority=None  Q=0 W  Q_nominal_specify=off  Q_nominal_value=1  Q_nominal_unit=W
  H : PMIOPort  Side=Left
  Q : PMIOPort  Port=2  Side=Left
  W : PMIOPort  Port=3  Side=Right
  T : PMIOPort  Port=4  Side=Right
  connections:
  Array of Thermal Nodes/RConn1 -- H/RConn1
  Qfrac/LConn1 -- Q/RConn1
  Qfrac/RConn1 -- AirMass/LConn1
  AirMass/LConn3 -- Wconv/LConn1
  Wconv/RConn1 -- W/RConn1
  AirMass/RConn1 -- T/RConn1
  Qconv1/LConn1 -- Array of Thermal Nodes/LConn10
  Qconv1/RConn1 -- Qconv2/RConn1 -- AirMass/LConn2 -- Qconv3/RConn1
  Qconv2/LConn1 -- Array of Thermal Nodes/LConn11
  Qconv3/LConn1 -- Array of Thermal Nodes/LConn12
  Array of Thermal Nodes/LConn1 -- Ins/LConn1 -- Array of Thermal Nodes/LConn2 -- Array of Thermal Nodes/LConn3 -- Array of Thermal Nodes/LConn4 -- Array of Thermal Nodes/LConn5 -- Array of Thermal Nodes/LConn6 -- Array of Thermal Nodes/LConn7 -- Array of Thermal Nodes/LConn8 -- Array of Thermal Nodes/LConn9

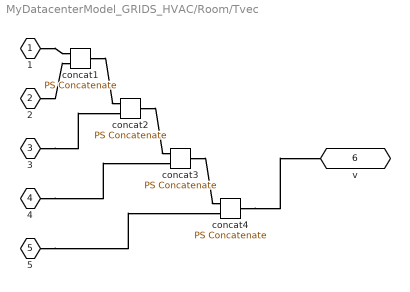
== system MyDatacenterModel_GRIDS_HVAC/Room/Tvec ==
  concat{1..4} (4 alike) : fl_lib/Physical Signals/Functions/PS Concatenate  catColumns=true
  1 : PMIOPort  Side=Left
  2 : PMIOPort  Port=2  Side=Left
  3 : PMIOPort  Port=3  Side=Left
  4 : PMIOPort  Port=4  Side=Left
  5 : PMIOPort  Port=5  Side=Left
  v : PMIOPort  Port=6  Side=Right
  connections:
  1/RConn1 -- concat1/LConn1
  2/RConn1 -- concat1/LConn2
  concat1/RConn1 -- concat2/LConn1
  3/RConn1 -- concat2/LConn2
  concat2/RConn1 -- concat3/LConn1
  4/RConn1 -- concat3/LConn2
  concat3/RConn1 -- concat4/LConn1
  5/RConn1 -- concat4/LConn2
  concat4/RConn1 -- v/RConn1

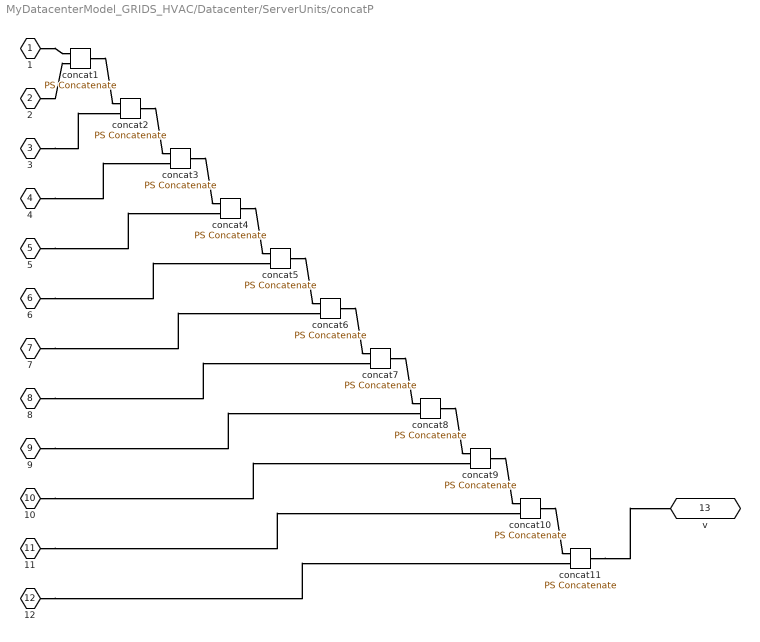
== system MyDatacenterModel_GRIDS_HVAC/Datacenter/ServerUnits/concatP ==
  concat{1..11} (11 alike) : fl_lib/Physical Signals/Functions/PS Concatenate  catColumns=true
  1 : PMIOPort  Side=Left
  2 : PMIOPort  Port=2  Side=Left
  3 : PMIOPort  Port=3  Side=Left
  4 : PMIOPort  Port=4  Side=Left
  5 : PMIOPort  Port=5  Side=Left
  6 : PMIOPort  Port=6  Side=Left
  7 : PMIOPort  Port=7  Side=Left
  8 : PMIOPort  Port=8  Side=Left
  9 : PMIOPort  Port=9  Side=Left
  10 : PMIOPort  Port=10  Side=Left
  11 : PMIOPort  Port=11  Side=Left
  12 : PMIOPort  Port=12  Side=Left
  v : PMIOPort  Port=13  Side=Right
  connections:
  1/RConn1 -- concat1/LConn1
  2/RConn1 -- concat1/LConn2
  concat1/RConn1 -- concat2/LConn1
  3/RConn1 -- concat2/LConn2
  concat2/RConn1 -- concat3/LConn1
  4/RConn1 -- concat3/LConn2
  concat3/RConn1 -- concat4/LConn1
  5/RConn1 -- concat4/LConn2
  concat4/RConn1 -- concat5/LConn1
  6/RConn1 -- concat5/LConn2
  concat5/RConn1 -- concat6/LConn1
  7/RConn1 -- concat6/LConn2
  concat6/RConn1 -- concat7/LConn1
  8/RConn1 -- concat7/LConn2
  concat7/RConn1 -- concat8/LConn1
  9/RConn1 -- concat8/LConn2
  concat8/RConn1 -- concat9/LConn1
  10/RConn1 -- concat9/LConn2
  concat9/RConn1 -- concat10/LConn1
  11/RConn1 -- concat10/LConn2
  concat10/RConn1 -- concat11/LConn1
  12/RConn1 -- concat11/LConn2
  concat11/RConn1 -- v/RConn1

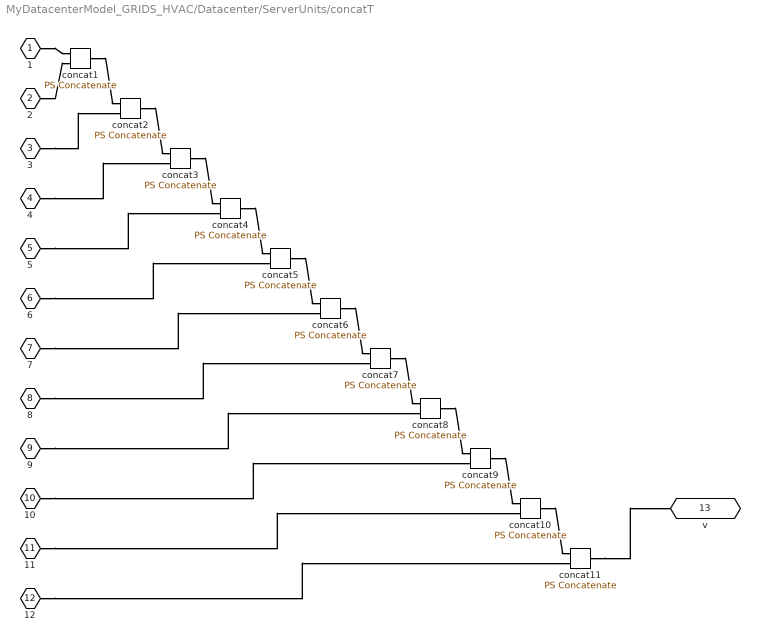
== system MyDatacenterModel_GRIDS_HVAC/Datacenter/ServerUnits/concatT ==
  concat{1..11} (11 alike) : fl_lib/Physical Signals/Functions/PS Concatenate  catColumns=true
  1 : PMIOPort  Side=Left
  2 : PMIOPort  Port=2  Side=Left
  3 : PMIOPort  Port=3  Side=Left
  4 : PMIOPort  Port=4  Side=Left
  5 : PMIOPort  Port=5  Side=Left
  6 : PMIOPort  Port=6  Side=Left
  7 : PMIOPort  Port=7  Side=Left
  8 : PMIOPort  Port=8  Side=Left
  9 : PMIOPort  Port=9  Side=Left
  10 : PMIOPort  Port=10  Side=Left
  11 : PMIOPort  Port=11  Side=Left
  12 : PMIOPort  Port=12  Side=Left
  v : PMIOPort  Port=13  Side=Right
  connections:
  1/RConn1 -- concat1/LConn1
  2/RConn1 -- concat1/LConn2
  concat1/RConn1 -- concat2/LConn1
  3/RConn1 -- concat2/LConn2
  concat2/RConn1 -- concat3/LConn1
  4/RConn1 -- concat3/LConn2
  concat3/RConn1 -- concat4/LConn1
  5/RConn1 -- concat4/LConn2
  concat4/RConn1 -- concat5/LConn1
  6/RConn1 -- concat5/LConn2
  concat5/RConn1 -- concat6/LConn1
  7/RConn1 -- concat6/LConn2
  concat6/RConn1 -- concat7/LConn1
  8/RConn1 -- concat7/LConn2
  concat7/RConn1 -- concat8/LConn1
  9/RConn1 -- concat8/LConn2
  concat8/RConn1 -- concat9/LConn1
  10/RConn1 -- concat9/LConn2
  concat9/RConn1 -- concat10/LConn1
  11/RConn1 -- concat10/LConn2
  concat10/RConn1 -- concat11/LConn1
  12/RConn1 -- concat11/LConn2
  concat11/RConn1 -- v/RConn1
